simulink model "selfmade_resonant_model"  (R2024b)
settings: Solver=ode45  StartTime=0.0  StopTime=sIn.simulation_time  MaxStep=0.001  RelTol=1e-3
values from neighbouring files (symbols this model uses):
  rads2rpm = 60/2/pi    (= 9.54929658551)    [load_params_resonant_case.m]
undefined symbols (not defined in the file or in its folder): daq, drv, gbox, mld, mot, PID, sens, sIn
libraries: simulink_extras x2
settings Model: Creator=Nihal  LastModifiedBy=Nihal

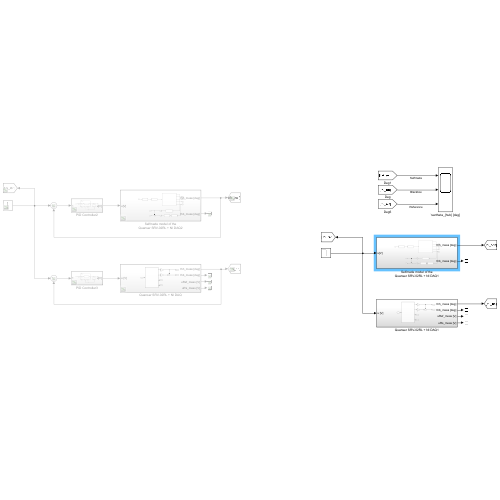
[thumbnail: Simulink's stored preview of the top-level diagram]
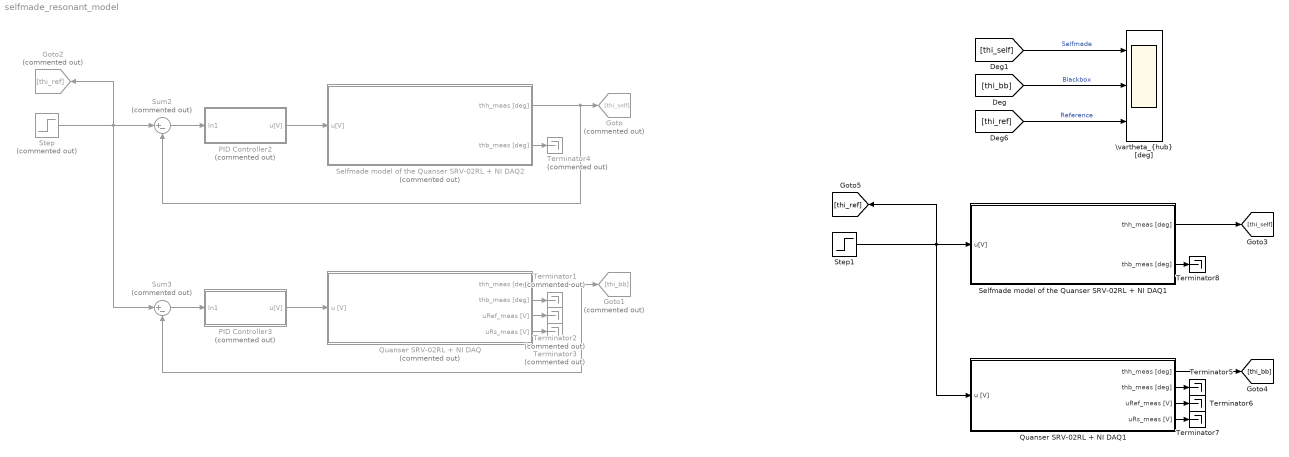
== system selfmade_resonant_model ==
  Goto : Goto  Commented=on  GotoTag=thi_self
  Goto1 : Goto  Commented=on  GotoTag=thi_bb
  Goto2 : Goto  Commented=on  GotoTag=thi_ref
  PID Controller2 : Subsystem  Commented=on
  PID Controller3 : Subsystem  Commented=on
  Quanser SRV-02RL + NI DAQ : Subsystem  Commented=on
  Quanser SRV-02RL + NI DAQ1 : Subsystem
  Selfmade model of the Quanser SRV-02RL + NI DAQ1 : Subsystem
  Selfmade model of the Quanser SRV-02RL + NI DAQ2 : Subsystem  Commented=on
  Step : Step  Commented=on  Time=sIn.step_time  After=sIn.position(2)  SampleTime=0
  Step1 : Step  Time=0.5  Before=1  After=0  SampleTime=1
  Sum2 : Sum  Commented=on  Inputs=|+-
  Sum3 : Sum  Commented=on  Inputs=|+-
  Terminator{1..4} (4 alike) : Terminator  Commented=on
  Terminator{5..8} (4 alike) : Terminator
  "\\vartheta_{hub} [deg]" : Scope  NumInputPorts=3
  wires:
  PID Controller2/1(u[V]) -> Selfmade model of the Quanser SRV-02RL + NI DAQ2/1(u[V])
  PID Controller3/1(u[V]) -> Quanser SRV-02RL + NI DAQ/1(u [V])
  Quanser SRV-02RL + NI DAQ/2(thb_meas [deg]) -> Terminator1/1
  Quanser SRV-02RL + NI DAQ/3(uRef_meas [V]) -> Terminator2/1
  Quanser SRV-02RL + NI DAQ/4(uRs_meas [V]) -> Terminator3/1
  Selfmade model of the Quanser SRV-02RL + NI DAQ2/2(thb_meas [deg]) -> Terminator4/1
  Sum2/1 -> PID Controller2/1(In1)
  Sum3/1 -> PID Controller3/1(In1)
  [thi_self] -> "\\vartheta_{hub} [deg]"/1  "Selfmade"
  [thi_ref] -> "\\vartheta_{hub} [deg]"/3  "Reference"
  [thi_bb] -> "\\vartheta_{hub} [deg]"/2  "Blackbox"
  Step/1 -> Goto2/1, Sum3/1, Sum2/1
  Selfmade model of the Quanser SRV-02RL + NI DAQ2/1(thh_meas [deg]) -> Goto/1, Sum2/2
  Quanser SRV-02RL + NI DAQ/1(thh_meas [deg]) -> Goto1/1, Sum3/2
  Selfmade model of the Quanser SRV-02RL + NI DAQ1/1(thh_meas [deg]) -> [thi_self]
  Quanser SRV-02RL + NI DAQ1/3(uRef_meas [V]) -> Terminator6/1
  Quanser SRV-02RL + NI DAQ1/4(uRs_meas [V]) -> Terminator7/1
  Quanser SRV-02RL + NI DAQ1/1(thh_meas [deg]) -> [thi_bb]
  Selfmade model of the Quanser SRV-02RL + NI DAQ1/2(thb_meas [deg]) -> Terminator8/1
  Quanser SRV-02RL + NI DAQ1/2(thb_meas [deg]) -> Terminator5/1
  Step1/1 -> Quanser SRV-02RL + NI DAQ1/1(u [V]), [thi_ref], Selfmade model of the Quanser SRV-02RL + NI DAQ1/1(u[V])

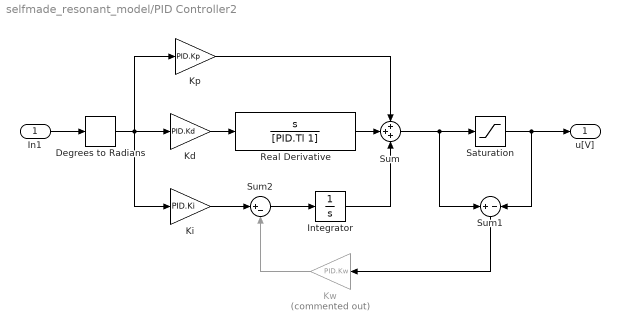
== system selfmade_resonant_model/PID Controller2 ==
  In1 : Inport
  Degrees to Radians : simulink_extras/Transformations/Degrees to Radians
  Integrator : Integrator
  Kd : Gain  Gain=PID.Kd
  Ki : Gain  Gain=PID.Ki
  Kp : Gain  Gain=PID.Kp
  Kw : Gain  Commented=on  Gain=PID.Kw
  Real Derivative : TransferFcn  Numerator=[1 0]  Denominator=[PID.Tl 1]
  Saturation : Saturate  UpperLimit=10  LowerLimit=-10
  Sum : Sum  Inputs=+++
  Sum1 : Sum  Inputs=+|-
  Sum2 : Sum  Inputs=|+-
  u[V] : Outport
  wires:
  In1/1 -> Degrees to Radians/1
  Sum/1 -> Sum1/1, Saturation/1
  Saturation/1 -> Sum1/2, u[V]/1
  Degrees to Radians/1 -> Ki/1, Kd/1, Kp/1
  Kd/1 -> Real Derivative/1
  Integrator/1 -> Sum/3
  Kp/1 -> Sum/1
  Real Derivative/1 -> Sum/2
  Ki/1 -> Sum2/1
  Sum2/1 -> Integrator/1
  Kw/1 -> Sum2/2
  Sum1/1 -> Kw/1

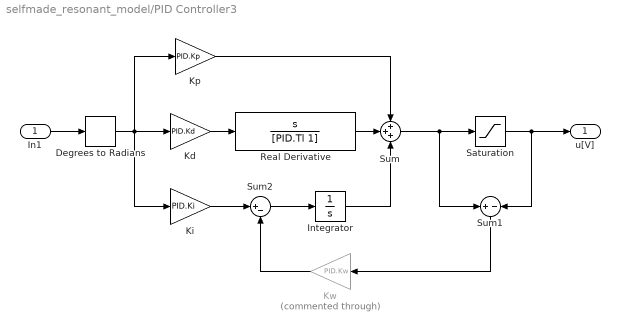
== system selfmade_resonant_model/PID Controller3 ==
  In1 : Inport
  Degrees to Radians : simulink_extras/Transformations/Degrees to Radians
  Integrator : Integrator
  Kd : Gain  Gain=PID.Kd
  Ki : Gain  Gain=PID.Ki
  Kp : Gain  Gain=PID.Kp
  Kw : Gain  Commented=through  Gain=PID.Kw
  Real Derivative : TransferFcn  Numerator=[1 0]  Denominator=[PID.Tl 1]
  Saturation : Saturate  UpperLimit=10  LowerLimit=-10
  Sum : Sum  Inputs=+++
  Sum1 : Sum  Inputs=+|-
  Sum2 : Sum  Inputs=|+-
  u[V] : Outport
  wires:
  In1/1 -> Degrees to Radians/1
  Sum/1 -> Sum1/1, Saturation/1
  Saturation/1 -> Sum1/2, u[V]/1
  Degrees to Radians/1 -> Ki/1, Kd/1, Kp/1
  Kd/1 -> Real Derivative/1
  Integrator/1 -> Sum/3
  Kp/1 -> Sum/1
  Real Derivative/1 -> Sum/2
  Ki/1 -> Sum2/1
  Sum2/1 -> Integrator/1
  Kw/1 -> Sum2/2
  Sum1/1 -> Kw/1

== system selfmade_resonant_model/Quanser SRV-02RL + NI DAQ ==
  u [V] : Inport
  Quanser SRV-02 + NI DAQ : Subsystem  mask(Quanser SRV-02 (with resonant load) + NI DAQ){Ts=0.001, fricType=Coulomb + viscous, lockShaft=off, beamInitPos=10}
      mask prompts: Ts "NI DAQ Sample Time:"; fricType "Friction model"; lockShaft "Lock motor shaft"; beamInitPos "Beam initial position [deg]:"
      mask help: Quanser SRV-02 (with resonant load) + NI DAQ model.
      mask init:
      | %%
      | % Riccardo Antonello (riccardo.antonello@unipd.it)
      | %
      | % April 28, 2020
      | %
      | % Dept. of Information Engineering, University of Padova
      | %
      | 
      | %%  Conversion gains
      | deg2rad = pi/180;                   %   [deg]   -> [rad]
      | rad2deg = 180/pi;                   %   [rad]   -> [deg]
      | 
      | 
      | %%  Sensors data
      | 
      | %   shunt resistor
      | sens.curr.Rs = 0.5;   
      | 
      | %   Hewlett-Packard HEDS-5540#A06 optical encoder
      | sens.enc.ppr = 500*4;                                                   %   pulses per rotation
      | sens.enc.pulse2deg = 360/sens.enc.ppr;                                  %   [pulses] -> [deg]
      | sens.enc.pulse2rad = 2*pi/sens.enc.ppr;                                 %   [pulses] -> [rad]
      | sens.enc.deg2pulse = sens.enc.ppr/360;                                  %   [deg] -> [pulses]
      | sens.enc.rad2pulse = sens.enc.ppr/2/pi;                                 %   [rad] -> [pulses]
      | 
      | %   potentiometer 2 (Spectrol 357-0-0-103) - installed on hub
      | sens.pot2.range.R      = 10e3;                                          %   ohmic value range 
      | sens.pot2.range.V      = 5;                                             %   voltage range
      | sens.pot2.range.th_deg = 340;                                           %   angle range [deg]
      | sens.pot2.range.th     = sens.pot2.range.th_deg * deg2rad;              %   angle range [rad]                           
      | sens.pot2.deg2V        = sens.pot2.range.V / sens.pot2.range.th_deg;    %   sensitivity [V/deg]
      | sens.pot2.rad2V        = sens.pot2.range.V / sens.pot2.range.th;        %   sensitivity [V/rad]
      | sens.pot2.V2deg        = 1/sens.pot2.deg2V;                             %   conversion gain [V] -> [deg]
      | sens.pot2.V2rad        = 1/sens.pot2.rad2V;                             %   conversion gain [V] -> [rad]
      | sens.pot2.noise.var    = 3.5e-7;                                        %   out noise variance [V^2]
      | 
      | 
      | %%  Data acquisition board (daq) data
      | 
      | %   NI PCI-6221 DAC data
      | daq.dac.bits = 16;                                  %   resolution (bits)
      | daq.dac.fs   = 10;                                  %   full scale 
      | daq.dac.q    = 2*daq.dac.fs/(2^daq.dac.bits-1);     %	quantization
      | 
      | %   NI PCI-6221 ADC data
      | daq.adc.bits = 16;                                  %   resolution (bits)
      | daq.adc.fs   = 10;                                  %   full scale (as set in SLDRT Analog Input block)
      | daq.adc.q    = 2*daq.adc.fs/(2^daq.adc.bits-1);     %   quantization   
      | 
      | 
      | %%  Set beam initial position
      | % SRV02Handle = find_system(gcb, ...
      | %     'LookUnderMasks', 'on', ...
      | %     'FindAll', 'on', ...
      | %     'FollowLinks', 'on', ...
      | %     'SearchDepth', '1', ...
      | %     'BlockType', 'ModelReference', ...
      | %     'Name', 'Quanser SRV-02');
      | %
      | % %get_param(SRV02Handle, 'InstanceParameters')
      | % InstanceParams = get_param(SRV02Handle, 'InstanceParameters');
      | % for k = 1:length(InstanceParams)
      | %     if strcmp(InstanceParams(k).Name, 'thb0')
      | %         if lockShaft
      | %             InstanceParams(k).Value = sprintf('%f', beamInitPos);
      | %         else
      | %             InstanceParams(k).Value = sprintf('%f', 0);    
      | %         end
      | %         set_param(SRV02Handle, 'InstanceParameters', InstanceParams);
      | %         break;
      | %     end
      | % end
      | 
      | if lockShaft
      |     thb0 = beamInitPos;
      | else
      |     thb0 = 0;    
      | end
      | 
      | 
      | %%  Mask initialization
      | if lockShaft
      |     
      |     %   find Inport handle
      |     InPortHandle = find_system(gcb, ...
      |         'LookUnderMasks', 'on', ...
      |         'FindAll', 'on', ...
      |         'FollowLinks', 'on', ...
      |         'SearchDepth', '1', ...
      |         'BlockType', 'Inport', ...
      |         'Name', 'u [V]');
      |     
      |     if ~isempty(InPortHandle)
      |     
      |         %   find DAC handle
      |         DACHandle = find_system(gcb, ...
      |             'LookUnderMasks', 'on', ...
      |             'FindAll', 'on', ...
      |             'FollowLinks', 'on', ...
      |             'SearchDepth', '1', ...
      |             'BlockType', 'SubSystem', ...
      |             'Name', 'DAC');  
      | 
      |         %   remove Inport output connection   
      |         InportConn = get_param(InPortHandle, 'PortConnectivity');
      |         delete_line(gcb, InportConn.Position);
      | 
      |         %   remove Inport block
      |         delete_block(InPortHandle);
      | 
      |         %   add Constant block
      |         ConstantHandle = add_block( ...
      |             'simulink/Sources/Constant', [gcb, '/u [V]'], ...
      |             'Position', [20   -37    50   -23], ...
      |             'Value', '0');
      | 
      |         %   connect Constant to DAC block
      |         DACPortHandles = get_param(DACHandle, 'PortHandles');
      |         ConstantPortHandles = get_param(ConstantHandle, 'PortHandles');
      |         add_line(gcb, ConstantPortHandles.Outport(1), DACPortHandles.Inport(1));
      |     
      |     end
      |     
      | else
      |     
      |     %   find Constant handle
      |     ConstantHandle = find_system(gcb, ...
      |         'LookUnderMasks', 'on', ...
      |         'FindAll', 'on', ...
      |         'FollowLinks', 'on', ...
      |         'SearchDepth', '1', ...
      |         'BlockType', 'Constant', ...
      |         'Name', 'u [V]');
      |     
      |     if ~isempty(ConstantHandle)
      |     
      |         %   find DAC handle
      |         DACHandle = find_system(gcb, ...
      |             'LookUnderMasks', 'on', ...
      |             'FindAll', 'on', ...
      |             'FollowLinks', 'on', ...
      |             'SearchDepth', '1', ...
      |             'BlockType', 'SubSystem', ...
      |             'Name', 'DAC');  
      |  
      |         %   remove Constant output connection   
      |         ConstantConn = get_param(ConstantHandle, 'PortConnectivity');
      |         delete_line(gcb, ConstantConn.Position);
      | 
      |         %   remove Inport block
      |         delete_block(ConstantHandle);   
      | 
      |         %   add Inport block
      |         InportHandle = add_block( ...
      |             'simulink/Sources/In1', [gcb, '/u [V]'], ...
      |             'Position', [20   -37    50   -23], ...
      |             'Port', '1');
      | 
      |         %   connect Constant to DAC block
      |         DACPortHandles = get_param(DACHandle, 'PortHandles');
      |         InportPortHandles = get_param(InportHandle, 'PortHandles');
      |         add_line(gcb, InportPortHandles.Outport(1), DACPortHandles.Inport(1));
      |     
      |      end
      |     
      | end
      mask Help:
      | Riccardo Antonello (antonello@dei.unipd.it)
      | 
      | April 28, 2020
      | 
      | Dept. of Information Engineering, University of Padova
      mask TypeOptions fricType: Coulomb + viscous | Karnopp
      mask Callback lockShaft:
      | %   get status of check box
      | lockShaft = get_param(gcb, 'lockShaft');
      | 
      | %   get current value of MaskVisibilities property
      | maskVisibilities = get_param(gcb, 'MaskVisibilities');
      | 
      | %   set visibility of the dialog box element
      | if strcmp(lockShaft, 'on')
      |     maskVisibilities{4} = 'on';
      | else
      |     maskVisibilities{4} = 'off';
      | end
      | 
      | % Set the 'MaskVisibilities' property for each parameter in mask
      | set_param( gcb, 'MaskVisibilities', maskVisibilities);
  Sum : Sum  Inputs=++|
  V2deg : Gain  Gain=sens.pot2.V2deg
  pulse2deg : Gain  Gain=sens.enc.pulse2deg
  thh_meas [deg] : Outport
  thb_meas [deg] : Outport  Port=2
  uRef_meas [V] : Outport  Port=3
  uRs_meas [V] : Outport  Port=4
  wires:
  Quanser SRV-02 + NI DAQ/2(uPot2_meas [V]) -> V2deg/1
  Sum/1 -> thb_meas [deg]/1
  pulse2deg/1 -> thh_meas [deg]/1, Sum/1
  V2deg/1 -> Sum/2
  Quanser SRV-02 + NI DAQ/1(thh_meas [pulses]) -> pulse2deg/1
  u [V]/1 -> Quanser SRV-02 + NI DAQ/1(u [V])
  Quanser SRV-02 + NI DAQ/3(uRef_meas [V]) -> uRef_meas [V]/1
  Quanser SRV-02 + NI DAQ/4(uRs_meas [V]) -> uRs_meas [V]/1

== system selfmade_resonant_model/Quanser SRV-02RL + NI DAQ1 ==
  u [V] : Inport
  Quanser SRV-02 + NI DAQ : Subsystem  mask(Quanser SRV-02 (with resonant load) + NI DAQ){Ts=0.001, fricType=Coulomb + viscous, lockShaft=off, beamInitPos=10}
      mask prompts: Ts "NI DAQ Sample Time:"; fricType "Friction model"; lockShaft "Lock motor shaft"; beamInitPos "Beam initial position [deg]:"
      mask help: Quanser SRV-02 (with resonant load) + NI DAQ model.
      mask init: same as selfmade_resonant_model/Quanser SRV-02RL + NI DAQ/Quanser SRV-02 + NI DAQ
      mask Help:
      | Riccardo Antonello (antonello@dei.unipd.it)
      | 
      | April 28, 2020
      | 
      | Dept. of Information Engineering, University of Padova
      mask TypeOptions fricType: Coulomb + viscous | Karnopp
      mask Callback lockShaft:
      | %   get status of check box
      | lockShaft = get_param(gcb, 'lockShaft');
      | 
      | %   get current value of MaskVisibilities property
      | maskVisibilities = get_param(gcb, 'MaskVisibilities');
      | 
      | %   set visibility of the dialog box element
      | if strcmp(lockShaft, 'on')
      |     maskVisibilities{4} = 'on';
      | else
      |     maskVisibilities{4} = 'off';
      | end
      | 
      | % Set the 'MaskVisibilities' property for each parameter in mask
      | set_param( gcb, 'MaskVisibilities', maskVisibilities);
  Sum : Sum  Inputs=++|
  V2deg : Gain  Gain=sens.pot2.V2deg
  pulse2deg : Gain  Gain=sens.enc.pulse2deg
  thh_meas [deg] : Outport
  thb_meas [deg] : Outport  Port=2
  uRef_meas [V] : Outport  Port=3
  uRs_meas [V] : Outport  Port=4
  wires:
  Quanser SRV-02 + NI DAQ/2(uPot2_meas [V]) -> V2deg/1
  Sum/1 -> thb_meas [deg]/1
  pulse2deg/1 -> thh_meas [deg]/1, Sum/1
  V2deg/1 -> Sum/2
  Quanser SRV-02 + NI DAQ/1(thh_meas [pulses]) -> pulse2deg/1
  u [V]/1 -> Quanser SRV-02 + NI DAQ/1(u [V])
  Quanser SRV-02 + NI DAQ/3(uRef_meas [V]) -> uRef_meas [V]/1
  Quanser SRV-02 + NI DAQ/4(uRs_meas [V]) -> uRs_meas [V]/1

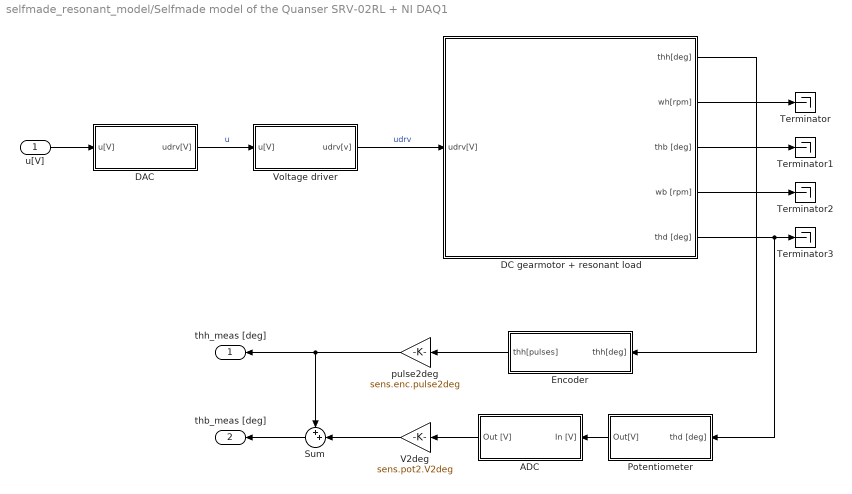
== system selfmade_resonant_model/Selfmade model of the Quanser SRV-02RL + NI DAQ1 ==
  u[V] : Inport
  ADC : Subsystem
  DAC : Subsystem
  DC gearmotor + resonant load : Subsystem
  Encoder : Subsystem
  Potentiometer : Subsystem
  Sum : Sum  Inputs=++|
  Terminator{,1..3} (4 alike) : Terminator
  V2deg : Gain  Gain=sens.pot2.V2deg
  Voltage driver : Subsystem
  pulse2deg : Gain  Gain=sens.enc.pulse2deg
  thh_meas [deg] : Outport
  thb_meas [deg] : Outport  Port=2
  wires:
  u[V]/1 -> DAC/1(u[V])
  DAC/1(udrv[V]) -> Voltage driver/1(u[V])  "u"
  Voltage driver/1(udrv[v]) -> DC gearmotor + resonant load/1(udrv[V])  "udrv"
  DC gearmotor + resonant load/1(thh[deg]) -> Encoder/1(thh[deg])
  Encoder/1(thh[pulses]) -> pulse2deg/1
  pulse2deg/1 -> Sum/1, thh_meas [deg]/1
  V2deg/1 -> Sum/2
  Sum/1 -> thb_meas [deg]/1
  DC gearmotor + resonant load/5(thd [deg]) -> Potentiometer/1(thd [deg]), Terminator3/1
  DC gearmotor + resonant load/4(wb [rpm]) -> Terminator2/1
  DC gearmotor + resonant load/3(thb [deg]) -> Terminator1/1
  DC gearmotor + resonant load/2(wh[rpm]) -> Terminator/1
  Potentiometer/1(Out[V]) -> ADC/1(In [V])
  ADC/1(Out [V]) -> V2deg/1

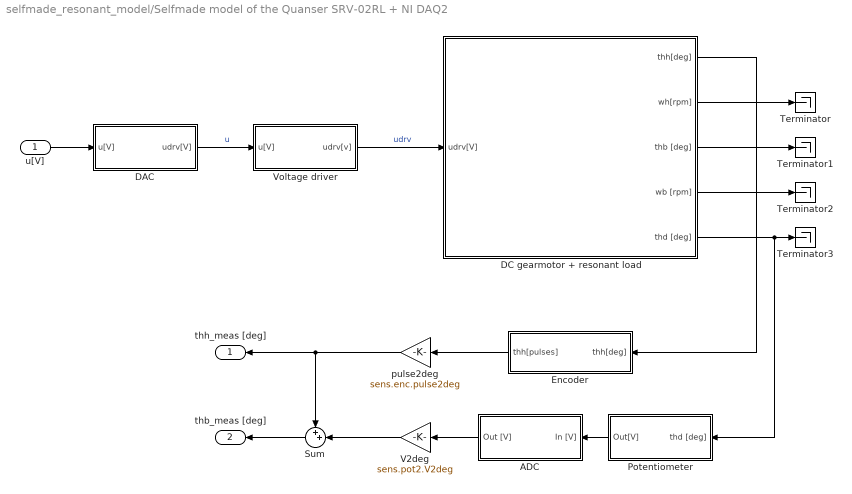
== system selfmade_resonant_model/Selfmade model of the Quanser SRV-02RL + NI DAQ2 ==
  u[V] : Inport
  ADC : Subsystem
  DAC : Subsystem
  DC gearmotor + resonant load : Subsystem
  Encoder : Subsystem
  Potentiometer : Subsystem
  Sum : Sum  Inputs=++|
  Terminator{,1..3} (4 alike) : Terminator
  V2deg : Gain  Gain=sens.pot2.V2deg
  Voltage driver : Subsystem
  pulse2deg : Gain  Gain=sens.enc.pulse2deg
  thh_meas [deg] : Outport
  thb_meas [deg] : Outport  Port=2
  wires:
  u[V]/1 -> DAC/1(u[V])
  DAC/1(udrv[V]) -> Voltage driver/1(u[V])  "u"
  Voltage driver/1(udrv[v]) -> DC gearmotor + resonant load/1(udrv[V])  "udrv"
  DC gearmotor + resonant load/1(thh[deg]) -> Encoder/1(thh[deg])
  Encoder/1(thh[pulses]) -> pulse2deg/1
  pulse2deg/1 -> Sum/1, thh_meas [deg]/1
  V2deg/1 -> Sum/2
  Sum/1 -> thb_meas [deg]/1
  DC gearmotor + resonant load/5(thd [deg]) -> Potentiometer/1(thd [deg]), Terminator3/1
  DC gearmotor + resonant load/4(wb [rpm]) -> Terminator2/1
  DC gearmotor + resonant load/3(thb [deg]) -> Terminator1/1
  DC gearmotor + resonant load/2(wh[rpm]) -> Terminator/1
  Potentiometer/1(Out[V]) -> ADC/1(In [V])
  ADC/1(Out [V]) -> V2deg/1

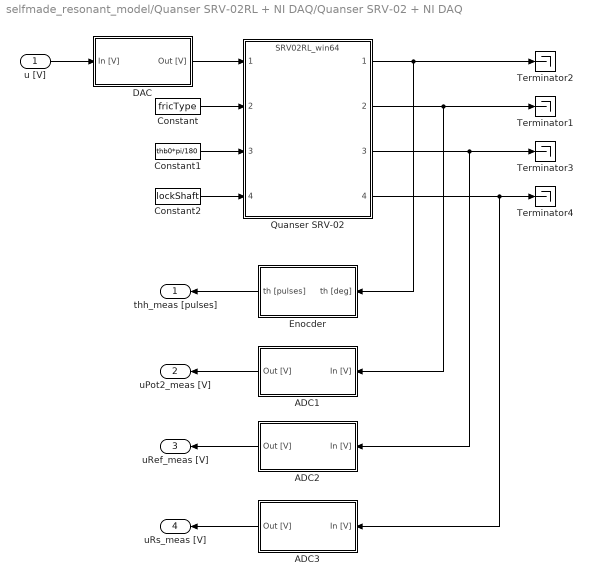
== system selfmade_resonant_model/Quanser SRV-02RL + NI DAQ/Quanser SRV-02 + NI DAQ ==
  u [V] : Inport
  ADC1 : Subsystem
  ADC2 : Subsystem
  ADC3 : Subsystem
  Constant : Constant  Value=fricType
  Constant1 : Constant  Value=thb0*pi/180  SampleTime=Inf
  Constant2 : Constant  Value=lockShaft  SampleTime=Inf
  DAC : Subsystem
  Enocder : Subsystem
  Quanser SRV-02 : ModelReference  ModelNameDialog=SRV02RL_win64.slxp  ModelReferenceVersion=1.76  CopyOfModelProtected=on
  Terminator{1..4} (4 alike) : Terminator
  thh_meas [pulses] : Outport
  uPot2_meas [V] : Outport  Port=2
  uRef_meas [V] : Outport  Port=3
  uRs_meas [V] : Outport  Port=4
  wires:
  Enocder/1(th [pulses]) -> thh_meas [pulses]/1
  ADC3/1(Out [V]) -> uRs_meas [V]/1
  DAC/1(Out [V]) -> Quanser SRV-02/1
  Quanser SRV-02/2 -> ADC1/1(In [V]), Terminator1/1
  Quanser SRV-02/1 -> Terminator2/1, Enocder/1(th [deg])
  Constant/1 -> Quanser SRV-02/2
  Quanser SRV-02/3 -> ADC2/1(In [V]), Terminator3/1
  ADC1/1(Out [V]) -> uPot2_meas [V]/1
  Constant1/1 -> Quanser SRV-02/3
  Constant2/1 -> Quanser SRV-02/4
  Quanser SRV-02/4 -> ADC3/1(In [V]), Terminator4/1
  ADC2/1(Out [V]) -> uRef_meas [V]/1
  u [V]/1 -> DAC/1(In [V])

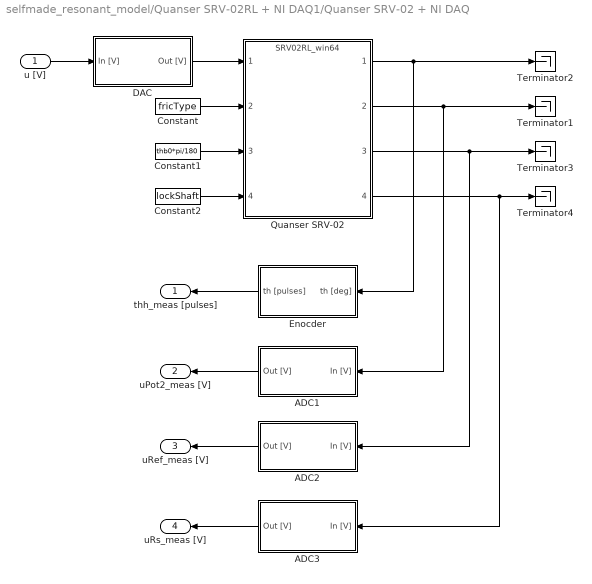
== system selfmade_resonant_model/Quanser SRV-02RL + NI DAQ1/Quanser SRV-02 + NI DAQ ==
  u [V] : Inport
  ADC1 : Subsystem
  ADC2 : Subsystem
  ADC3 : Subsystem
  Constant : Constant  Value=fricType
  Constant1 : Constant  Value=thb0*pi/180  SampleTime=Inf
  Constant2 : Constant  Value=lockShaft  SampleTime=Inf
  DAC : Subsystem
  Enocder : Subsystem
  Quanser SRV-02 : ModelReference  ModelNameDialog=SRV02RL_win64.slxp  ModelReferenceVersion=1.76  CopyOfModelProtected=on
  Terminator{1..4} (4 alike) : Terminator
  thh_meas [pulses] : Outport
  uPot2_meas [V] : Outport  Port=2
  uRef_meas [V] : Outport  Port=3
  uRs_meas [V] : Outport  Port=4
  wires:
  Enocder/1(th [pulses]) -> thh_meas [pulses]/1
  ADC3/1(Out [V]) -> uRs_meas [V]/1
  DAC/1(Out [V]) -> Quanser SRV-02/1
  Quanser SRV-02/2 -> ADC1/1(In [V]), Terminator1/1
  Quanser SRV-02/1 -> Terminator2/1, Enocder/1(th [deg])
  Constant/1 -> Quanser SRV-02/2
  Quanser SRV-02/3 -> ADC2/1(In [V]), Terminator3/1
  ADC1/1(Out [V]) -> uPot2_meas [V]/1
  Constant1/1 -> Quanser SRV-02/3
  Constant2/1 -> Quanser SRV-02/4
  Quanser SRV-02/4 -> ADC3/1(In [V]), Terminator4/1
  ADC2/1(Out [V]) -> uRef_meas [V]/1
  u [V]/1 -> DAC/1(In [V])

== system selfmade_resonant_model/Selfmade model of the Quanser SRV-02RL + NI DAQ1/ADC ==
  In [V] : Inport
  ADC Sampling : ZeroOrderHold  SampleTime=daq.adc.Ts
  ADC Saturation : Saturate  UpperLimit=2.5  LowerLimit=-2.5
  ADC quantization : Quantizer  QuantizationInterval=daq.adc.q
  Out [V] : Outport
  wires:
  In [V]/1 -> ADC Sampling/1
  ADC Sampling/1 -> ADC quantization/1
  ADC quantization/1 -> ADC Saturation/1
  ADC Saturation/1 -> Out [V]/1

== system selfmade_resonant_model/Selfmade model of the Quanser SRV-02RL + NI DAQ1/DAC ==
  u[V] : Inport
  Quantizer : Quantizer  QuantizationInterval=daq.dac.q
  Saturation : Saturate  UpperLimit=10  LowerLimit=-10
  Zero-Order Hold : ZeroOrderHold  SampleTime=1e-3
  udrv[V] : Outport
  wires:
  Zero-Order Hold/1 -> Quantizer/1
  u[V]/1 -> Zero-Order Hold/1
  Quantizer/1 -> Saturation/1
  Saturation/1 -> udrv[V]/1

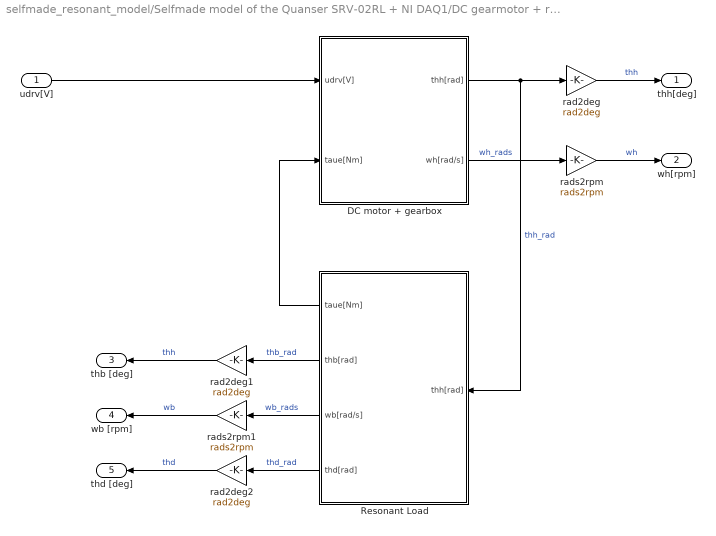
== system selfmade_resonant_model/Selfmade model of the Quanser SRV-02RL + NI DAQ1/DC gearmotor + resonant load ==
  udrv[V] : Inport
  DC motor + gearbox : Subsystem
  Resonant Load : Subsystem
  rad2deg : Gain  Gain=rad2deg
  rad2deg1 : Gain  Gain=rad2deg
  rad2deg2 : Gain  Gain=rad2deg
  rads2rpm : Gain  Gain=rads2rpm
  rads2rpm1 : Gain  Gain=rads2rpm
  thh[deg] : Outport
  wh[rpm] : Outport  Port=2
  thb [deg] : Outport  Port=3
  wb [rpm] : Outport  Port=4
  thd [deg] : Outport  Port=5
  wires:
  DC motor + gearbox/1(thh[rad]) -> Resonant Load/1(thh[rad]), rad2deg/1  "thh_rad"
  Resonant Load/2(thb[rad]) -> rad2deg1/1  "thb_rad"
  rad2deg2/1 -> thd [deg]/1  "thd"
  rad2deg/1 -> thh[deg]/1  "thh"
  Resonant Load/4(thd[rad]) -> rad2deg2/1  "thd_rad"
  Resonant Load/1(taue[Nm]) -> DC motor + gearbox/2(taue[Nm])
  rad2deg1/1 -> thb [deg]/1  "thh"
  rads2rpm1/1 -> wb [rpm]/1  "wb"
  Resonant Load/3(wb[rad/s]) -> rads2rpm1/1  "wb_rads"
  DC motor + gearbox/2(wh[rad/s]) -> rads2rpm/1  "wh_rads"
  rads2rpm/1 -> wh[rpm]/1  "wh"
  udrv[V]/1 -> DC motor + gearbox/1(udrv[V])

== system selfmade_resonant_model/Selfmade model of the Quanser SRV-02RL + NI DAQ1/Encoder ==
  thh[deg] : Inport
  Gain : Gain  Gain=1/sens.enc.pulse2deg
  Quantizer : Quantizer  QuantizationInterval=sens.enc.pulse2deg
  Zero-Order Hold : ZeroOrderHold  SampleTime=1e-3
  thh[pulses] : Outport
  wires:
  thh[deg]/1 -> Zero-Order Hold/1
  Gain/1 -> thh[pulses]/1
  Quantizer/1 -> Gain/1
  Zero-Order Hold/1 -> Quantizer/1

== system selfmade_resonant_model/Selfmade model of the Quanser SRV-02RL + NI DAQ1/Potentiometer ==
  thd [deg] : Inport
  Sensor output noise [V] : RandomNumber  Variance=sens.pot2.noise.var  SampleTime=daq.adc.Ts
  Sum : Sum  Inputs=|++
  deg2V : Gain  Gain=sens.pot2.deg2V
  Out[V] : Outport
  wires:
  thd [deg]/1 -> deg2V/1
  deg2V/1 -> Sum/1
  Sensor output noise [V]/1 -> Sum/2
  Sum/1 -> Out[V]/1

== system selfmade_resonant_model/Selfmade model of the Quanser SRV-02RL + NI DAQ1/Voltage driver ==
  u[V] : Inport
  Saturation : Saturate  UpperLimit=12  LowerLimit=-12
  Transfer Fcn : TransferFcn  Numerator=[drv.dcgain]  Denominator=[drv.Tc 1]
  udrv[v] : Outport
  wires:
  u[V]/1 -> Transfer Fcn/1
  Transfer Fcn/1 -> Saturation/1
  Saturation/1 -> udrv[v]/1

== system selfmade_resonant_model/Selfmade model of the Quanser SRV-02RL + NI DAQ2/ADC ==
  In [V] : Inport
  ADC Sampling : ZeroOrderHold  SampleTime=daq.adc.Ts
  ADC Saturation : Saturate  UpperLimit=2.5  LowerLimit=-2.5
  ADC quantization : Quantizer  QuantizationInterval=daq.adc.q
  Out [V] : Outport
  wires:
  In [V]/1 -> ADC Sampling/1
  ADC Sampling/1 -> ADC quantization/1
  ADC quantization/1 -> ADC Saturation/1
  ADC Saturation/1 -> Out [V]/1

== system selfmade_resonant_model/Selfmade model of the Quanser SRV-02RL + NI DAQ2/DAC ==
  u[V] : Inport
  Quantizer : Quantizer  QuantizationInterval=daq.dac.q
  Saturation : Saturate  UpperLimit=10  LowerLimit=-10
  Zero-Order Hold : ZeroOrderHold  SampleTime=1e-3
  udrv[V] : Outport
  wires:
  Zero-Order Hold/1 -> Quantizer/1
  u[V]/1 -> Zero-Order Hold/1
  Quantizer/1 -> Saturation/1
  Saturation/1 -> udrv[V]/1

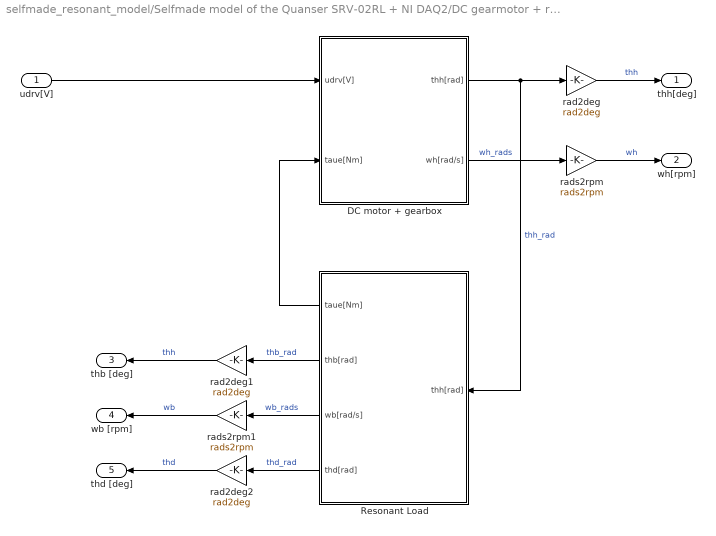
== system selfmade_resonant_model/Selfmade model of the Quanser SRV-02RL + NI DAQ2/DC gearmotor + resonant load ==
  udrv[V] : Inport
  DC motor + gearbox : Subsystem
  Resonant Load : Subsystem
  rad2deg : Gain  Gain=rad2deg
  rad2deg1 : Gain  Gain=rad2deg
  rad2deg2 : Gain  Gain=rad2deg
  rads2rpm : Gain  Gain=rads2rpm
  rads2rpm1 : Gain  Gain=rads2rpm
  thh[deg] : Outport
  wh[rpm] : Outport  Port=2
  thb [deg] : Outport  Port=3
  wb [rpm] : Outport  Port=4
  thd [deg] : Outport  Port=5
  wires:
  DC motor + gearbox/1(thh[rad]) -> Resonant Load/1(thh[rad]), rad2deg/1  "thh_rad"
  Resonant Load/2(thb[rad]) -> rad2deg1/1  "thb_rad"
  rad2deg2/1 -> thd [deg]/1  "thd"
  rad2deg/1 -> thh[deg]/1  "thh"
  Resonant Load/4(thd[rad]) -> rad2deg2/1  "thd_rad"
  Resonant Load/1(taue[Nm]) -> DC motor + gearbox/2(taue[Nm])
  rad2deg1/1 -> thb [deg]/1  "thh"
  rads2rpm1/1 -> wb [rpm]/1  "wb"
  Resonant Load/3(wb[rad/s]) -> rads2rpm1/1  "wb_rads"
  DC motor + gearbox/2(wh[rad/s]) -> rads2rpm/1  "wh_rads"
  rads2rpm/1 -> wh[rpm]/1  "wh"
  udrv[V]/1 -> DC motor + gearbox/1(udrv[V])

== system selfmade_resonant_model/Selfmade model of the Quanser SRV-02RL + NI DAQ2/Encoder ==
  thh[deg] : Inport
  Gain : Gain  Gain=1/sens.enc.pulse2deg
  Quantizer : Quantizer  QuantizationInterval=sens.enc.pulse2deg
  Zero-Order Hold : ZeroOrderHold  SampleTime=1e-3
  thh[pulses] : Outport
  wires:
  thh[deg]/1 -> Zero-Order Hold/1
  Gain/1 -> thh[pulses]/1
  Quantizer/1 -> Gain/1
  Zero-Order Hold/1 -> Quantizer/1

== system selfmade_resonant_model/Selfmade model of the Quanser SRV-02RL + NI DAQ2/Potentiometer ==
  thd [deg] : Inport
  Sensor output noise [V] : RandomNumber  Variance=sens.pot2.noise.var  SampleTime=daq.adc.Ts
  Sum : Sum  Inputs=|++
  deg2V : Gain  Gain=sens.pot2.deg2V
  Out[V] : Outport
  wires:
  thd [deg]/1 -> deg2V/1
  deg2V/1 -> Sum/1
  Sensor output noise [V]/1 -> Sum/2
  Sum/1 -> Out[V]/1

== system selfmade_resonant_model/Selfmade model of the Quanser SRV-02RL + NI DAQ2/Voltage driver ==
  u[V] : Inport
  Saturation : Saturate  UpperLimit=12  LowerLimit=-12
  Transfer Fcn : TransferFcn  Numerator=[drv.dcgain]  Denominator=[drv.Tc 1]
  udrv[v] : Outport
  wires:
  u[V]/1 -> Transfer Fcn/1
  Transfer Fcn/1 -> Saturation/1
  Saturation/1 -> udrv[v]/1

== system selfmade_resonant_model/Quanser SRV-02RL + NI DAQ/Quanser SRV-02 + NI DAQ/ADC1 ==
  In [V] : Inport
  ADC quantization : Quantizer  QuantizationInterval=daq.adc.q
  ADC sampling : ZeroOrderHold  SampleTime=Ts
  ADC saturation : Saturate  UpperLimit=daq.adc.fs  LowerLimit=-daq.adc.fs
  Out [V] : Outport
  wires:
  ADC saturation/1 -> Out [V]/1
  ADC sampling/1 -> ADC quantization/1
  In [V]/1 -> ADC sampling/1
  ADC quantization/1 -> ADC saturation/1

== system selfmade_resonant_model/Quanser SRV-02RL + NI DAQ/Quanser SRV-02 + NI DAQ/ADC2 ==
  In [V] : Inport
  ADC quantization : Quantizer  QuantizationInterval=daq.adc.q
  ADC sampling : ZeroOrderHold  SampleTime=Ts
  ADC saturation : Saturate  UpperLimit=daq.adc.fs  LowerLimit=-daq.adc.fs
  Out [V] : Outport
  wires:
  ADC quantization/1 -> ADC saturation/1
  In [V]/1 -> ADC sampling/1
  ADC sampling/1 -> ADC quantization/1
  ADC saturation/1 -> Out [V]/1

== system selfmade_resonant_model/Quanser SRV-02RL + NI DAQ/Quanser SRV-02 + NI DAQ/ADC3 ==
  In [V] : Inport
  Quantizer : Quantizer  QuantizationInterval=daq.adc.q
  Saturation : Saturate  UpperLimit=daq.adc.fs  LowerLimit=-daq.adc.fs
  Zero-Order Hold : ZeroOrderHold  SampleTime=Ts
  Out [V] : Outport
  wires:
  Saturation/1 -> Out [V]/1
  In [V]/1 -> Zero-Order Hold/1
  Quantizer/1 -> Saturation/1
  Zero-Order Hold/1 -> Quantizer/1

== system selfmade_resonant_model/Quanser SRV-02RL + NI DAQ/Quanser SRV-02 + NI DAQ/DAC ==
  In [V] : Inport
  Quantizer : Quantizer  QuantizationInterval=daq.dac.q
  Saturation : Saturate  UpperLimit=daq.dac.fs  LowerLimit=-daq.dac.fs
  Zero-Order Hold : ZeroOrderHold  SampleTime=Ts
  Out [V] : Outport
  wires:
  Quantizer/1 -> Saturation/1
  In [V]/1 -> Zero-Order Hold/1
  Zero-Order Hold/1 -> Quantizer/1
  Saturation/1 -> Out [V]/1

== system selfmade_resonant_model/Quanser SRV-02RL + NI DAQ/Quanser SRV-02 + NI DAQ/Enocder ==
  th [deg] : Inport
  Quantizer : Quantizer  QuantizationInterval=sens.enc.pulse2deg
  Zero-Order Hold : ZeroOrderHold  SampleTime=Ts
  deg2pulse : Gain  Gain=sens.enc.deg2pulse
  th [pulses] : Outport
  wires:
  Quantizer/1 -> deg2pulse/1
  th [deg]/1 -> Zero-Order Hold/1
  Zero-Order Hold/1 -> Quantizer/1
  deg2pulse/1 -> th [pulses]/1

== system selfmade_resonant_model/Quanser SRV-02RL + NI DAQ1/Quanser SRV-02 + NI DAQ/ADC1 ==
  In [V] : Inport
  ADC quantization : Quantizer  QuantizationInterval=daq.adc.q
  ADC sampling : ZeroOrderHold  SampleTime=Ts
  ADC saturation : Saturate  UpperLimit=daq.adc.fs  LowerLimit=-daq.adc.fs
  Out [V] : Outport
  wires:
  ADC saturation/1 -> Out [V]/1
  ADC sampling/1 -> ADC quantization/1
  In [V]/1 -> ADC sampling/1
  ADC quantization/1 -> ADC saturation/1

== system selfmade_resonant_model/Quanser SRV-02RL + NI DAQ1/Quanser SRV-02 + NI DAQ/ADC2 ==
  In [V] : Inport
  ADC quantization : Quantizer  QuantizationInterval=daq.adc.q
  ADC sampling : ZeroOrderHold  SampleTime=Ts
  ADC saturation : Saturate  UpperLimit=daq.adc.fs  LowerLimit=-daq.adc.fs
  Out [V] : Outport
  wires:
  ADC quantization/1 -> ADC saturation/1
  In [V]/1 -> ADC sampling/1
  ADC sampling/1 -> ADC quantization/1
  ADC saturation/1 -> Out [V]/1

== system selfmade_resonant_model/Quanser SRV-02RL + NI DAQ1/Quanser SRV-02 + NI DAQ/ADC3 ==
  In [V] : Inport
  Quantizer : Quantizer  QuantizationInterval=daq.adc.q
  Saturation : Saturate  UpperLimit=daq.adc.fs  LowerLimit=-daq.adc.fs
  Zero-Order Hold : ZeroOrderHold  SampleTime=Ts
  Out [V] : Outport
  wires:
  Saturation/1 -> Out [V]/1
  In [V]/1 -> Zero-Order Hold/1
  Quantizer/1 -> Saturation/1
  Zero-Order Hold/1 -> Quantizer/1

== system selfmade_resonant_model/Quanser SRV-02RL + NI DAQ1/Quanser SRV-02 + NI DAQ/DAC ==
  In [V] : Inport
  Quantizer : Quantizer  QuantizationInterval=daq.dac.q
  Saturation : Saturate  UpperLimit=daq.dac.fs  LowerLimit=-daq.dac.fs
  Zero-Order Hold : ZeroOrderHold  SampleTime=Ts
  Out [V] : Outport
  wires:
  Quantizer/1 -> Saturation/1
  In [V]/1 -> Zero-Order Hold/1
  Zero-Order Hold/1 -> Quantizer/1
  Saturation/1 -> Out [V]/1

== system selfmade_resonant_model/Quanser SRV-02RL + NI DAQ1/Quanser SRV-02 + NI DAQ/Enocder ==
  th [deg] : Inport
  Quantizer : Quantizer  QuantizationInterval=sens.enc.pulse2deg
  Zero-Order Hold : ZeroOrderHold  SampleTime=Ts
  deg2pulse : Gain  Gain=sens.enc.deg2pulse
  th [pulses] : Outport
  wires:
  Quantizer/1 -> deg2pulse/1
  th [deg]/1 -> Zero-Order Hold/1
  Zero-Order Hold/1 -> Quantizer/1
  deg2pulse/1 -> th [pulses]/1

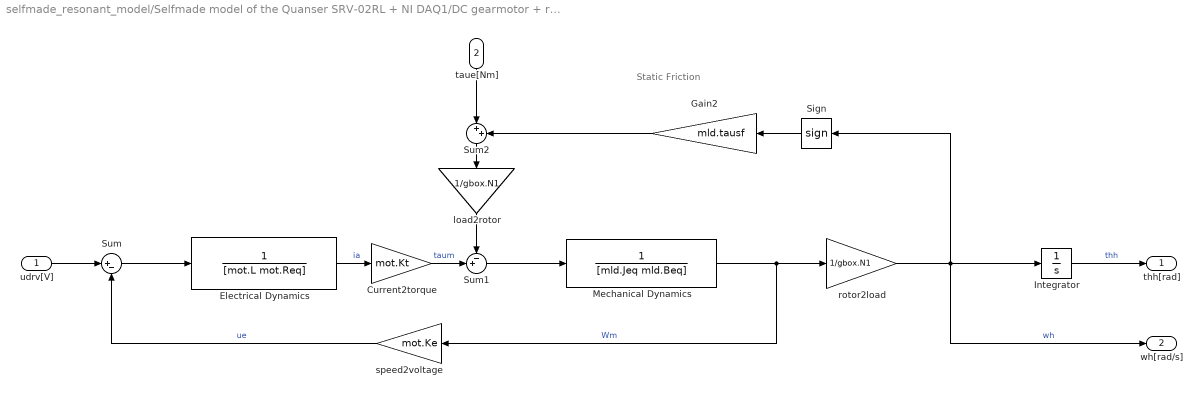
== system selfmade_resonant_model/Selfmade model of the Quanser SRV-02RL + NI DAQ1/DC gearmotor + resonant load/DC motor + gearbox ==
  note: Static Friction
  udrv[V] : Inport
  taue[Nm] : Inport  Port=2
  Current2torque : Gain  Gain=mot.Kt
  Electrical Dynamics : TransferFcn  Denominator=[mot.L mot.Req]
  Gain2 : Gain  Gain=mld.tausf
  Integrator : Integrator
  Mechanical Dynamics : TransferFcn  Denominator=[mld.Jeq mld.Beq]
  Sign : Signum  ZeroCross=off
  Sum : Sum  Inputs=|+-
  Sum1 : Sum  Inputs=-+|
  Sum2 : Sum  Inputs=|++
  load2rotor : Gain  Gain=1/gbox.N1
  rotor2load : Gain  Gain=1/gbox.N1
  speed2voltage : Gain  Gain=mot.Ke
  thh[rad] : Outport
  wh[rad/s] : Outport  Port=2
  wires:
  udrv[V]/1 -> Sum/1
  Sum/1 -> Electrical Dynamics/1
  Electrical Dynamics/1 -> Current2torque/1  "ia"
  load2rotor/1 -> Sum1/1
  Sign/1 -> Gain2/1
  Mechanical Dynamics/1 -> speed2voltage/1, rotor2load/1  "Wm"
  rotor2load/1 -> wh[rad/s]/1, Sign/1, Integrator/1  "wh"
  Sum1/1 -> Mechanical Dynamics/1
  Current2torque/1 -> Sum1/2  "taum"
  speed2voltage/1 -> Sum/2  "ue"
  Integrator/1 -> thh[rad]/1  "thh"
  taue[Nm]/1 -> Sum2/1
  Sum2/1 -> load2rotor/1
  Gain2/1 -> Sum2/2

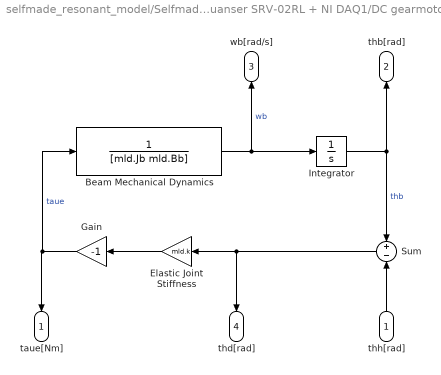
== system selfmade_resonant_model/Selfmade model of the Quanser SRV-02RL + NI DAQ1/DC gearmotor + resonant load/Resonant Load ==
  thh[rad] : Inport
  Beam Mechanical Dynamics : TransferFcn  Denominator=[mld.Jb mld.Bb]
  Elastic Joint Stiffness : Gain  Gain=mld.k
  Gain : Gain  Gain=-1
  Integrator : Integrator
  Sum : Sum  Inputs=+|-
  taue[Nm] : Outport
  thb[rad] : Outport  Port=2
  wb[rad/s] : Outport  Port=3
  thd[rad] : Outport  Port=4
  wires:
  thh[rad]/1 -> Sum/2
  Integrator/1 -> Sum/1, thb[rad]/1  "thb"
  Sum/1 -> thd[rad]/1, Elastic Joint Stiffness/1
  Elastic Joint Stiffness/1 -> Gain/1
  Gain/1 -> Beam Mechanical Dynamics/1, taue[Nm]/1  "taue"
  Beam Mechanical Dynamics/1 -> wb[rad/s]/1, Integrator/1  "wb"

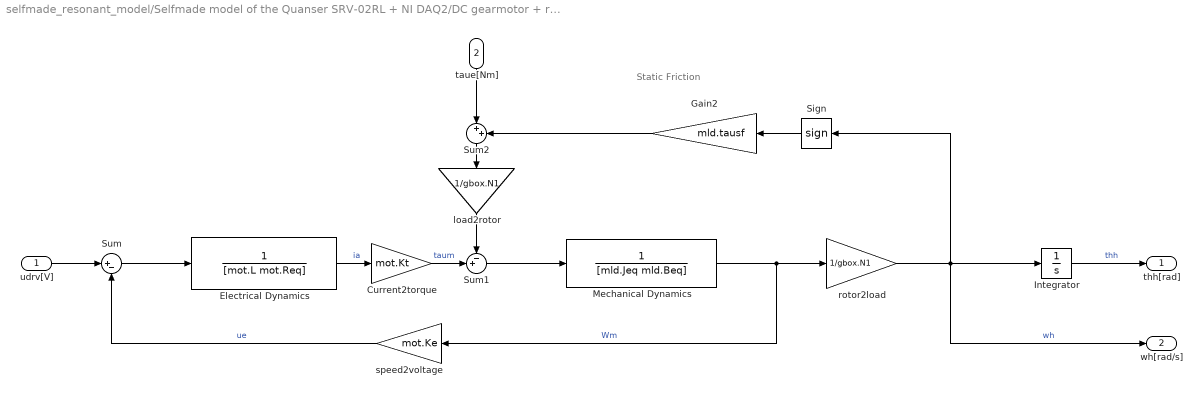
== system selfmade_resonant_model/Selfmade model of the Quanser SRV-02RL + NI DAQ2/DC gearmotor + resonant load/DC motor + gearbox ==
  note: Static Friction
  udrv[V] : Inport
  taue[Nm] : Inport  Port=2
  Current2torque : Gain  Gain=mot.Kt
  Electrical Dynamics : TransferFcn  Denominator=[mot.L mot.Req]
  Gain2 : Gain  Gain=mld.tausf
  Integrator : Integrator
  Mechanical Dynamics : TransferFcn  Denominator=[mld.Jeq mld.Beq]
  Sign : Signum  ZeroCross=off
  Sum : Sum  Inputs=|+-
  Sum1 : Sum  Inputs=-+|
  Sum2 : Sum  Inputs=|++
  load2rotor : Gain  Gain=1/gbox.N1
  rotor2load : Gain  Gain=1/gbox.N1
  speed2voltage : Gain  Gain=mot.Ke
  thh[rad] : Outport
  wh[rad/s] : Outport  Port=2
  wires:
  udrv[V]/1 -> Sum/1
  Sum/1 -> Electrical Dynamics/1
  Electrical Dynamics/1 -> Current2torque/1  "ia"
  load2rotor/1 -> Sum1/1
  Sign/1 -> Gain2/1
  Mechanical Dynamics/1 -> speed2voltage/1, rotor2load/1  "Wm"
  rotor2load/1 -> wh[rad/s]/1, Sign/1, Integrator/1  "wh"
  Sum1/1 -> Mechanical Dynamics/1
  Current2torque/1 -> Sum1/2  "taum"
  speed2voltage/1 -> Sum/2  "ue"
  Integrator/1 -> thh[rad]/1  "thh"
  taue[Nm]/1 -> Sum2/1
  Sum2/1 -> load2rotor/1
  Gain2/1 -> Sum2/2

== system selfmade_resonant_model/Selfmade model of the Quanser SRV-02RL + NI DAQ2/DC gearmotor + resonant load/Resonant Load ==
  thh[rad] : Inport
  Beam Mechanical Dynamics : TransferFcn  Denominator=[mld.Jb mld.Bb]
  Elastic Joint Stiffness : Gain  Gain=mld.K
  Gain : Gain  Gain=-1
  Integrator : Integrator
  Sum : Sum  Inputs=+|-
  taue[Nm] : Outport
  thb[rad] : Outport  Port=2
  wb[rad/s] : Outport  Port=3
  thd[rad] : Outport  Port=4
  wires:
  thh[rad]/1 -> Sum/2
  Integrator/1 -> Sum/1, thb[rad]/1  "thb"
  Sum/1 -> thd[rad]/1, Elastic Joint Stiffness/1
  Elastic Joint Stiffness/1 -> Gain/1
  Gain/1 -> Beam Mechanical Dynamics/1, taue[Nm]/1  "taue"
  Beam Mechanical Dynamics/1 -> wb[rad/s]/1, Integrator/1  "wb"
